simulink model "simulation"  (R2022b)
settings: Solver=VariableStepAuto  StartTime=0.0  StopTime=10.0  RelTol=1e-3
InitFcn:
  | awake;
undefined symbols (not defined in the file or in its folder): d, g, J, L, m, R
settings Model: Creator=onuru  LastModifiedBy=onuru

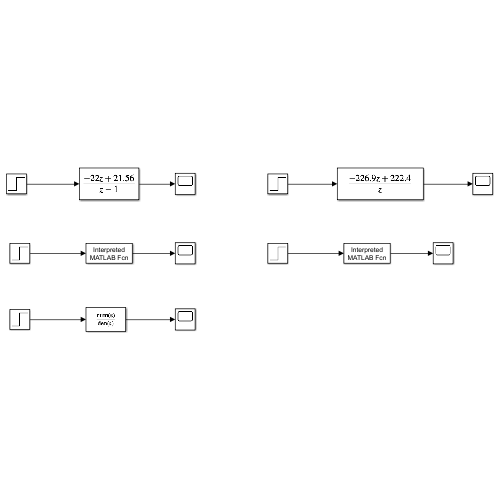
[thumbnail: Simulink's stored preview of the top-level diagram]
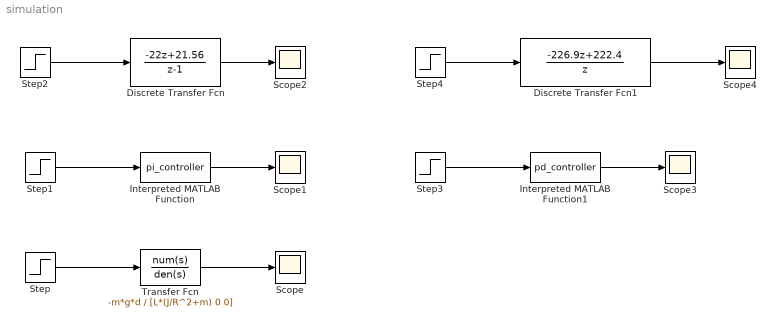
== system simulation ==
  Discrete Transfer Fcn : DiscreteTransferFcn  Numerator=[-22 21.56]  Denominator=[1 -1]  SampleTime=.1
  Discrete Transfer Fcn1 : DiscreteTransferFcn  Numerator=[-226.9 222.4]  Denominator=[1 0]  SampleTime=.1
  Interpreted MATLAB Function : MATLABFcn  MATLABFcn=pi_controller
  Interpreted MATLAB Function1 : MATLABFcn  MATLABFcn=pd_controller
  Scope{,1..4} (5 alike) : Scope
  Step : Step  SampleTime=0
  Step{1..4} (4 alike) : Step  Time=0  After=.3  SampleTime=0
  Transfer Fcn : TransferFcn  Numerator=-m*g*d  Denominator=[L*(J/R^2+m) 0 0]
  wires:
  Transfer Fcn/1 -> Scope/1
  Step/1 -> Transfer Fcn/1
  Interpreted MATLAB Function/1 -> Scope1/1
  Step1/1 -> Interpreted MATLAB Function/1
  Step2/1 -> Discrete Transfer Fcn/1
  Discrete Transfer Fcn/1 -> Scope2/1
  Interpreted MATLAB Function1/1 -> Scope3/1
  Step3/1 -> Interpreted MATLAB Function1/1
  Step4/1 -> Discrete Transfer Fcn1/1
  Discrete Transfer Fcn1/1 -> Scope4/1
